simulink model "Batch_Model"  (Simulink 8.3)
settings: Solver=ode15s  StartTime=0.0  StopTime=10.0  RelTol=1e-2
values from neighbouring files (symbols this model uses):
  a0 = 555.556    [Ann_Main.m]    (also in Main_Program.m)
  B1 = 0.193    [Ann_Main.m]    (also in Main_Program.m)
  B2 = 0.167    [Ann_Main.m]    (also in Main_Program.m)
  c = S_Out    (= 0)    [Ann_Main.m]    (also in Main_Program.m = S_Out)
  c0 = 5.2*10^-5    (= 5.2e-05)    [Ann_Main.m]    (also in Main_Program.m)
  c1 = 16.4    [Ann_Main.m]    (also in Main_Program.m)
  c2 = 2.3    [Ann_Main.m]    (also in Main_Program.m)
  c3 = 1.563    [Ann_Main.m]    (also in Main_Program.m)
  CpC = 4.187    [Ann_Main.m]    (also in Main_Program.m)
  CpM = 1.675    [Ann_Main.m]    (also in Main_Program.m)
  CpP = 3.140    (= 3.14)    [Ann_Main.m]    (also in Main_Program.m)
  CpW = 4.187    [Ann_Main.m]    (also in Main_Program.m)
  d0 = 0.814    [Ann_Main.m]    (also in Main_Program.m)
  d1 = -5.13    [Ann_Main.m]    (also in Main_Program.m)
  deltaH = 70152.16    [Ann_Main.m]    (also in Main_Program.m)
  E = 29560.89    [Ann_Main.m]    (also in Main_Program.m)
  hf = 0.704    [Ann_Main.m]    (also in Main_Program.m = 0)
  i = 1.2    [Ann_Main.m]    (also in Main_Program.m)
  k0 = 55    [Ann_Main.m]    (also in Main_Program.m)
  k1 = 1000    [Ann_Main.m]    (also in Main_Program.m)
  k2 = 0.4    [Ann_Main.m]    (also in Main_Program.m)
  ki = 1    [Ann_Main.m]    (also in Main_Program.m = 0.8)
  mC = 21.455    [Ann_Main.m]    (also in Main_Program.m)
  mC_r = 0.9412    [Ann_Main.m]    (also in Main_Program.m)
  mMin = 0    [Ann_Main.m]    (also in Main_Program.m)
  mW = 42.750    (= 42.75)    [Ann_Main.m]    (also in Main_Program.m)
  MWM = 104.0    (= 104)    [Ann_Main.m]    (also in Main_Program.m)
  P = 1.594    [Ann_Main.m]    (also in Main_Program.m; S_ControllerPID.m = error-spid.error1)
  R = 8.314    [Ann_Main.m]    (also in Main_Program.m)
  rhoM = 900.0    (= 900)    [Ann_Main.m]    (also in Main_Program.m)
  rhoP = 1040.0    (= 1040)    [Ann_Main.m]    (also in Main_Program.m)
  rhoW = 1000.0    (= 1000)    [Ann_Main.m]    (also in Main_Program.m)
  TAmb = 305.38    [Ann_Main.m]    (also in Main_Program.m)
  tauP = 40.2    [Ann_Main.m]    (also in Main_Program.m)
  theta1 = 22.8    [Ann_Main.m]    (also in Main_Program.m)
  theta2 = 15    [Ann_Main.m]    (also in Main_Program.m)
  Tinlet = 294.26    [Ann_Main.m]    (also in Main_Program.m)
  TM = TAmb    (= 305.38)    [Ann_Main.m]    (also in Main_Program.m)
  Tsteam = 449.82    [Ann_Main.m]    (also in Main_Program.m)
  UAloss = 0.00567567    [Ann_Main.m]    (also in Main_Program.m)
settings Model: Creator=lijin  LastModifiedBy=Administrator
settings DataIOCC: ExternalInput=[k',mMin',c']
settings OptimizationCC: ExpressionDepthLimit=2147483647
settings DebuggingCC: FcnCallInpInsideContextMsg=UseLocalSettings

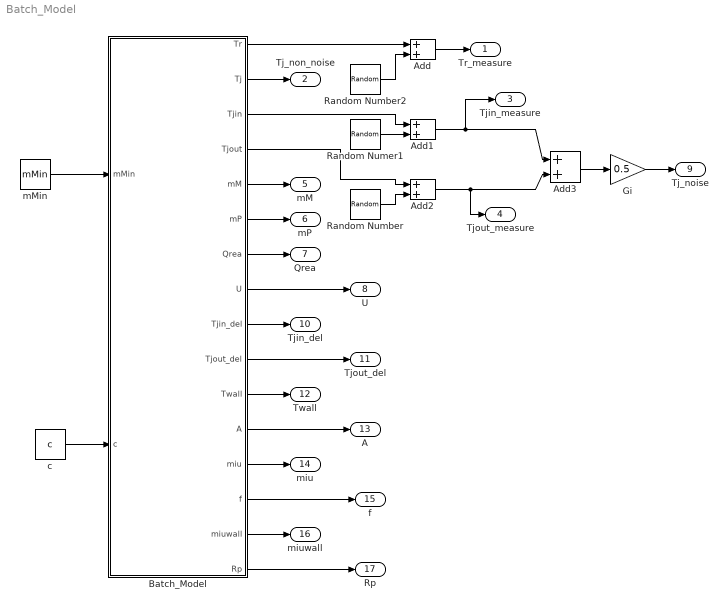
== system Batch_Model ==
  Add{,1..3} (4 alike) : Sum
  Batch_Model : Subsystem
  Gi : Gain  Gain=0.5
  Random Number : RandomNumber  Variance=0.01  Seed=34  SampleTime=0.1
  Random Number2 : RandomNumber  Variance=0.01  Seed=56  SampleTime=0.1
  Random Numer1 : RandomNumber  Variance=0.01  Seed=23  SampleTime=0.1
  c : Constant  Value=c  OutMin=[0]  OutMax=[100]  LockScale=on
  mMin : Constant  Value=mMin  OutMin=[0]  OutMax=[100]  LockScale=on
  Tr_measure : Outport
  Tj_non_noise : Outport  Port=2
  Tjin_measure : Outport  Port=3
  Tjout_measure : Outport  Port=4
  mM : Outport  Port=5
  mP : Outport  Port=6
  Qrea : Outport  Port=7
  U : Outport  Port=8
  Tj_noise : Outport  Port=9
  Tjin_del : Outport  Port=10
  Tjout_del : Outport  Port=11
  Twall : Outport  Port=12
  A : Outport  Port=13
  miu : Outport  Port=14
  f : Outport  Port=15
  miuwall : Outport  Port=16
  Rp : Outport  Port=17
  wires:
  mMin/1 -> Batch_Model/1(mMin)
  c/1 -> Batch_Model/2(c)
  Batch_Model/8(U) -> U/1
  Batch_Model/7(Qrea) -> Qrea/1
  Batch_Model/6(mP) -> mP/1
  Batch_Model/5(mM) -> mM/1
  Batch_Model/2(Tj) -> Tj_non_noise/1
  Batch_Model/3(Tjin) -> Add1/1
  Batch_Model/4(Tjout) -> Add2/1
  Random Numer1/1 -> Add1/2
  Random Number/1 -> Add2/2
  Batch_Model/1(Tr) -> Add/1
  Random Number2/1 -> Add/2
  Add/1 -> Tr_measure/1
  Add1/1 -> Tjin_measure/1, Add3/1
  Add2/1 -> Tjout_measure/1, Add3/2
  Add3/1 -> Gi/1
  Gi/1 -> Tj_noise/1
  Batch_Model/9(Tjin_del) -> Tjin_del/1
  Batch_Model/10(Tjout_del) -> Tjout_del/1
  Batch_Model/11(Twall) -> Twall/1
  Batch_Model/12(A) -> A/1
  Batch_Model/13(miu) -> miu/1
  Batch_Model/14(f) -> f/1
  Batch_Model/15(miuwall) -> miuwall/1
  Batch_Model/16(Rp) -> Rp/1

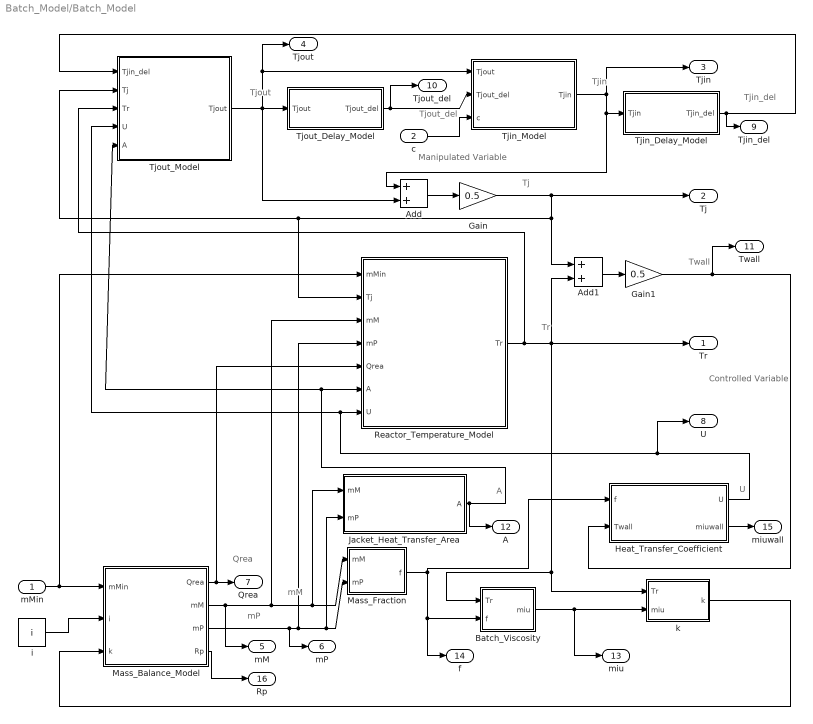
== system Batch_Model/Batch_Model ==
  note: Tj
  note: Tr
  note: Tjout
  note: Tjin
  note: Tjout_del
  note: Tjin_del
  note: U
  note: A
  note: mP
  note: mM
  note: Qrea
  note: Manipulated Variable
  note: Controlled Variable
  note: Twall
  mMin : Inport
  c : Inport  Port=2
  Add : Sum
  Add1 : Sum
  Batch_Viscosity : Subsystem
  Gain : Gain  Gain=0.5
  Gain1 : Gain  Gain=0.5
  Heat_Transfer_Coefficient : Subsystem
  Jacket_Heat_Transfer_Area : Subsystem
  Mass_Balance_Model : Subsystem
  Mass_Fraction : Subsystem
  Reactor_Temperature_Model : Subsystem
  Tjin_Delay_Model : Subsystem
  Tjin_Model : Subsystem
  Tjout_Delay_Model : Subsystem
  Tjout_Model : Subsystem
  i : Constant  Value=i
  k : Subsystem
  Tr : Outport
  Tj : Outport  Port=2
  Tjin : Outport  Port=3
  Tjout : Outport  Port=4
  mM : Outport  Port=5
  mP : Outport  Port=6
  Qrea : Outport  Port=7
  U : Outport  Port=8
  Tjin_del : Outport  Port=9
  Tjout_del : Outport  Port=10
  Twall : Outport  Port=11
  A : Outport  Port=12
  miu : Outport  Port=13
  f : Outport  Port=14
  miuwall : Outport  Port=15
  Rp : Outport  Port=16
  wires:
  Mass_Balance_Model/2(mM) -> Mass_Fraction/1(mM), Jacket_Heat_Transfer_Area/1(mM), Reactor_Temperature_Model/3(mM), mM/1
  Mass_Balance_Model/3(mP) -> Mass_Fraction/2(mP), Jacket_Heat_Transfer_Area/2(mP), Reactor_Temperature_Model/4(mP), mP/1
  Mass_Fraction/1(f) -> Batch_Viscosity/2(f), f/1, Heat_Transfer_Coefficient/1(f)
  Batch_Viscosity/1(miu) -> k/2(miu), miu/1
  Jacket_Heat_Transfer_Area/1(A) -> Reactor_Temperature_Model/6(A), Tjout_Model/5(A), A/1
  Heat_Transfer_Coefficient/1(U) -> Tjout_Model/4(U), Reactor_Temperature_Model/7(U), U/1
  Mass_Balance_Model/1(Qrea) -> Qrea/1, Reactor_Temperature_Model/5(Qrea)
  Tjout_Model/1(Tjout) -> Tjout_Delay_Model/1(Tjout), Tjout/1, Tjin_Model/1(Tjout), Add/2
  Tjout_Delay_Model/1(Tjout_del) -> Tjin_Model/2(Tjout_del), Tjout_del/1
  c/1 -> Tjin_Model/3(c)
  Tjin_Model/1(Tjin) -> Tjin_Delay_Model/1(Tjin), Add/1, Tjin/1
  Tjin_Delay_Model/1(Tjin_del) -> Tjout_Model/1(Tjin_del), Tjin_del/1
  Add/1 -> Gain/1
  Gain/1 -> Add1/1, Reactor_Temperature_Model/2(Tj), Tjout_Model/2(Tj), Tj/1
  mMin/1 -> Reactor_Temperature_Model/1(mMin), Mass_Balance_Model/1(mMin)
  Reactor_Temperature_Model/1(Tr) -> Tr/1, k/1(Tr), Batch_Viscosity/1(Tr), Add1/2, Tjout_Model/3(Tr)
  Add1/1 -> Gain1/1
  Gain1/1 -> Heat_Transfer_Coefficient/2(Twall), Twall/1
  Heat_Transfer_Coefficient/2(miuwall) -> miuwall/1
  Mass_Balance_Model/4(Rp) -> Rp/1
  i/1 -> Mass_Balance_Model/2(i)
  k/1(k) -> Mass_Balance_Model/3(k)

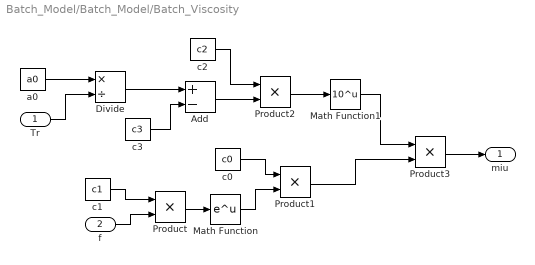
== system Batch_Model/Batch_Model/Batch_Viscosity ==
  Tr : Inport
  f : Inport  Port=2
  Add : Sum  Inputs=+-
  Divide : Product  Inputs=*/
  Math Function : Math  SaturateOnIntegerOverflow=on
  Math Function1 : Math  Operator=10^u  SaturateOnIntegerOverflow=on
  Product{,1..3} (4 alike) : Product  RndMeth=Zero
  a0 : Constant  Value=a0
  c0 : Constant  Value=c0
  c1 : Constant  Value=c1
  c2 : Constant  Value=c2
  c3 : Constant  Value=c3
  miu : Outport
  wires:
  c1/1 -> Product/1
  f/1 -> Product/2
  Product/1 -> Math Function/1
  Math Function/1 -> Product1/2
  c0/1 -> Product1/1
  a0/1 -> Divide/1
  Tr/1 -> Divide/2
  Divide/1 -> Add/1
  c3/1 -> Add/2
  Add/1 -> Product2/2
  c2/1 -> Product2/1
  Product2/1 -> Math Function1/1
  Math Function1/1 -> Product3/1
  Product1/1 -> Product3/2
  Product3/1 -> miu/1

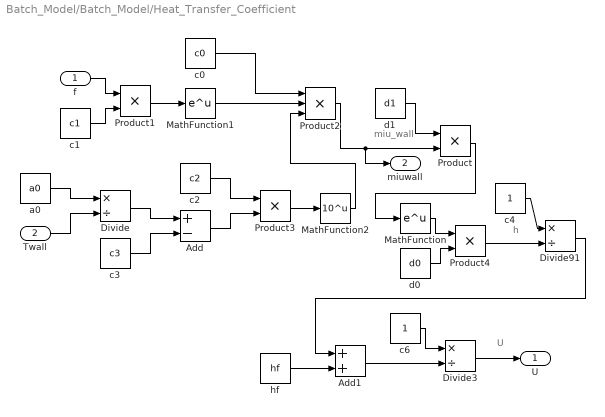
== system Batch_Model/Batch_Model/Heat_Transfer_Coefficient ==
  note: miu_wall
  note: h
  note: U
  f : Inport
  Twall : Inport  Port=2
  Add : Sum  Inputs=+-
  Add1 : Sum
  Divide : Product  Inputs=*/
  Divide3 : Product  Inputs=*/
  Divide91 : Product  Inputs=*/
  MathFunction : Math  SaturateOnIntegerOverflow=on
  MathFunction1 : Math  SaturateOnIntegerOverflow=on
  MathFunction2 : Math  Operator=10^u  SaturateOnIntegerOverflow=on
  Product{,1,3..4} (4 alike) : Product  RndMeth=Zero
  Product2 : Product  Inputs=3  RndMeth=Zero
  a0 : Constant  Value=a0
  c0 : Constant  Value=c0
  c1 : Constant  Value=c1
  c2 : Constant  Value=c2
  c3 : Constant  Value=c3
  c4 : Constant
  c6 : Constant
  d0 : Constant  Value=d0
  d1 : Constant  Value=d1
  hf : Constant  Value=hf
  U : Outport
  miuwall : Outport  Port=2
  wires:
  f/1 -> Product1/1
  c1/1 -> Product1/2
  Product1/1 -> MathFunction1/1
  a0/1 -> Divide/1
  Twall/1 -> Divide/2
  c3/1 -> Add/2
  Divide/1 -> Add/1
  Add/1 -> Product3/2
  c2/1 -> Product3/1
  Product3/1 -> MathFunction2/1
  c0/1 -> Product2/1
  MathFunction1/1 -> Product2/2
  MathFunction2/1 -> Product2/3
  Product2/1 -> Product/2, miuwall/1
  d1/1 -> Product/1
  MathFunction/1 -> Product4/1
  d0/1 -> Product4/2
  Product/1 -> MathFunction/1
  c4/1 -> Divide91/1
  Divide91/1 -> Add1/1
  c6/1 -> Divide3/1
  Add1/1 -> Divide3/2
  Divide3/1 -> U/1
  hf/1 -> Add1/2
  Product4/1 -> Divide91/2

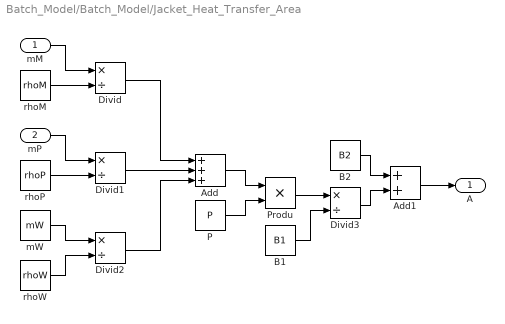
== system Batch_Model/Batch_Model/Jacket_Heat_Transfer_Area ==
  mM : Inport
  mP : Inport  Port=2
  Add : Sum  Inputs=+++
  Add1 : Sum
  B1 : Constant  Value=B1
  B2 : Constant  Value=B2
  Divid{,1..3} (4 alike) : Product  Inputs=*/
  P : Constant  Value=P
  Produ : Product  RndMeth=Zero
  mW : Constant  Value=mW
  rhoM : Constant  Value=rhoM
  rhoP : Constant  Value=rhoP
  rhoW : Constant  Value=rhoW
  A : Outport
  wires:
  mM/1 -> Divid/1
  rhoM/1 -> Divid/2
  mP/1 -> Divid1/1
  rhoP/1 -> Divid1/2
  mW/1 -> Divid2/1
  rhoW/1 -> Divid2/2
  Divid/1 -> Add/1
  Divid1/1 -> Add/2
  Divid2/1 -> Add/3
  Add/1 -> Produ/1
  P/1 -> Produ/2
  Produ/1 -> Divid3/1
  B1/1 -> Divid3/2
  B2/1 -> Add1/1
  Divid3/1 -> Add1/2
  Add1/1 -> A/1

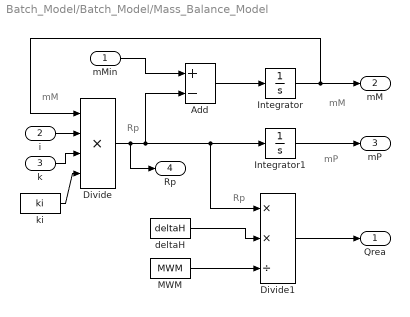
== system Batch_Model/Batch_Model/Mass_Balance_Model ==
  note: mM
  note: Rp
  note: Rp
  note: mM
  note: mP
  mMin : Inport
  i : Inport  Port=2
  k : Inport  Port=3
  Add : Sum  Inputs=+-
  Divide : Product  Inputs=****
  Divide1 : Product  Inputs=**/
  Integrator : Integrator
  Integrator1 : Integrator
  MWM : Constant  Value=MWM
  deltaH : Constant  Value=deltaH
  ki : Constant  Value=ki
  Qrea : Outport
  mM : Outport  Port=2
  mP : Outport  Port=3
  Rp : Outport  Port=4
  wires:
  i/1 -> Divide/2
  k/1 -> Divide/3
  mMin/1 -> Add/1
  Divide/1 -> Integrator1/1, Divide1/1, Add/2, Rp/1
  Add/1 -> Integrator/1
  Integrator/1 -> Divide/1, mM/1
  Integrator1/1 -> mP/1
  deltaH/1 -> Divide1/2
  Divide1/1 -> Qrea/1
  MWM/1 -> Divide1/3
  ki/1 -> Divide/4

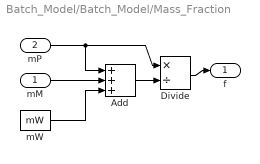
== system Batch_Model/Batch_Model/Mass_Fraction ==
  mM : Inport
  mP : Inport  Port=2
  Add : Sum  Inputs=+++
  Divide : Product  Inputs=*/
  mW : Constant  Value=mW
  f : Outport
  wires:
  mW/1 -> Add/3
  mM/1 -> Add/2
  mP/1 -> Add/1, Divide/1
  Add/1 -> Divide/2
  Divide/1 -> f/1

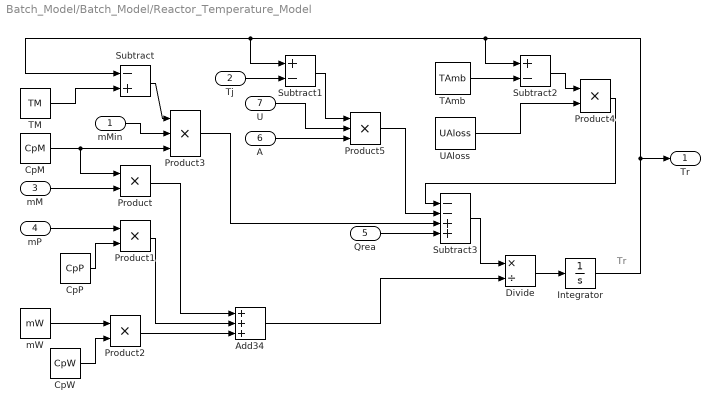
== system Batch_Model/Batch_Model/Reactor_Temperature_Model ==
  note: Tr
  mMin : Inport
  Tj : Inport  Port=2
  mM : Inport  Port=3
  mP : Inport  Port=4
  Qrea : Inport  Port=5
  A : Inport  Port=6
  U : Inport  Port=7
  Add34 : Sum  Inputs=+++
  CpM : Constant  Value=CpM
  CpP : Constant  Value=CpP
  CpW : Constant  Value=CpW
  Divide : Product  Inputs=*/
  Integrator : Integrator
  Product{,1..2,4} (4 alike) : Product  RndMeth=Zero
  Product3 : Product  Inputs=3  RndMeth=Zero
  Product5 : Product  Inputs=3  RndMeth=Zero
  Subtract : Sum  Inputs=-+
  Subtract1 : Sum  Inputs=+-
  Subtract2 : Sum  Inputs=+-
  Subtract3 : Sum  Inputs=--++
  TAmb : Constant  Value=TAmb
  TM : Constant  Value=TM
  UAloss : Constant  Value=UAloss
  mW : Constant  Value=mW
  Tr : Outport
  wires:
  mP/1 -> Product1/1
  CpP/1 -> Product1/2
  mW/1 -> Product2/1
  CpW/1 -> Product2/2
  Product/1 -> Add34/1
  Product1/1 -> Add34/2
  Product2/1 -> Add34/3
  mM/1 -> Product/2
  CpM/1 -> Product/1, Product3/3
  Tj/1 -> Subtract1/2
  mMin/1 -> Product3/2
  Subtract/1 -> Product3/1
  A/1 -> Product5/3
  U/1 -> Product5/2
  Subtract1/1 -> Product5/1
  TAmb/1 -> Subtract2/2
  Subtract2/1 -> Product4/1
  UAloss/1 -> Product4/2
  Integrator/1 -> Tr/1, Subtract/1, Subtract1/1, Subtract2/1
  Product4/1 -> Subtract3/1
  Product5/1 -> Subtract3/2
  Product3/1 -> Subtract3/3
  Qrea/1 -> Subtract3/4
  Subtract3/1 -> Divide/1
  Add34/1 -> Divide/2
  Divide/1 -> Integrator/1
  TM/1 -> Subtract/2

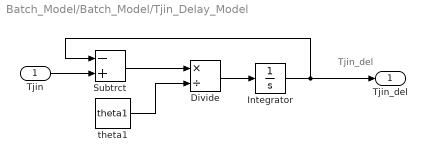
== system Batch_Model/Batch_Model/Tjin_Delay_Model ==
  note: Tjin_del
  Tjin : Inport
  Divide : Product  Inputs=*/
  Integrator : Integrator
  Subtrct : Sum  Inputs=-+
  theta1 : Constant  Value=theta1
  Tjin_del : Outport
  wires:
  Subtrct/1 -> Divide/1
  theta1/1 -> Divide/2
  Tjin/1 -> Subtrct/2
  Divide/1 -> Integrator/1
  Integrator/1 -> Tjin_del/1, Subtrct/1

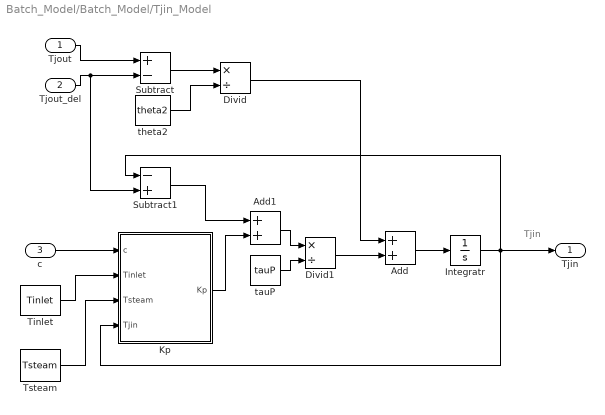
== system Batch_Model/Batch_Model/Tjin_Model ==
  note: Tjin
  Tjout : Inport
  Tjout_del : Inport  Port=2
  c : Inport  Port=3
  Add : Sum
  Add1 : Sum
  Divid : Product  Inputs=*/
  Divid1 : Product  Inputs=*/
  Integratr : Integrator
  Kp : MATLAB Function  TreatAsAtomicUnit=on
  Subtract : Sum  Inputs=+-
  Subtract1 : Sum  Inputs=-+
  Tinlet : Constant  Value=Tinlet
  Tsteam : Constant  Value=Tsteam
  tauP : Constant  Value=tauP
  theta2 : Constant  Value=theta2
  Tjin : Outport
  wires:
  Tjout/1 -> Subtract/1
  Tjout_del/1 -> Subtract/2, Subtract1/2
  Subtract/1 -> Divid/1
  theta2/1 -> Divid/2
  c/1 -> Kp/1(c)
  Tsteam/1 -> Kp/3(Tsteam)
  Integratr/1 -> Tjin/1, Subtract1/1, Kp/4(Tjin)
  Subtract1/1 -> Add1/1
  Add1/1 -> Divid1/1
  tauP/1 -> Divid1/2
  Divid/1 -> Add/1
  Divid1/1 -> Add/2
  Add/1 -> Integratr/1
  Kp/1(Kp) -> Add1/2
  Tinlet/1 -> Kp/2(Tinlet)

== system Batch_Model/Batch_Model/Tjout_Delay_Model ==
  note: Tjout_del
  Tjout : Inport
  Divide : Product  Inputs=*/
  Integrator : Integrator
  Subtrct : Sum  Inputs=-+
  theta2 : Constant  Value=theta2
  Tjout_del : Outport
  wires:
  Subtrct/1 -> Divide/1
  theta2/1 -> Divide/2
  Tjout/1 -> Subtrct/2
  Divide/1 -> Integrator/1
  Integrator/1 -> Tjout_del/1, Subtrct/1

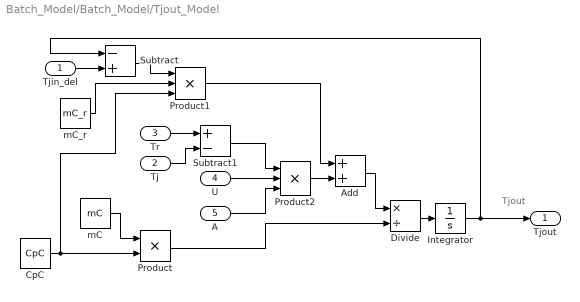
== system Batch_Model/Batch_Model/Tjout_Model ==
  note: Tjout
  Tjin_del : Inport
  Tj : Inport  Port=2
  Tr : Inport  Port=3
  U : Inport  Port=4
  A : Inport  Port=5
  Add : Sum
  CpC : Constant  Value=CpC
  Divide : Product  Inputs=*/
  Integrator : Integrator
  Product : Product  RndMeth=Zero
  Product1 : Product  Inputs=3  RndMeth=Zero
  Product2 : Product  Inputs=3  RndMeth=Zero
  Subtract : Sum  Inputs=-+
  Subtract1 : Sum  Inputs=+-
  mC : Constant  Value=mC
  mC_r : Constant  Value=mC_r
  Tjout : Outport
  wires:
  mC_r/1 -> Product1/2
  Tjin_del/1 -> Subtract/2
  Subtract/1 -> Product1/1
  Tr/1 -> Subtract1/1
  Tj/1 -> Subtract1/2
  Subtract1/1 -> Product2/1
  U/1 -> Product2/2
  A/1 -> Product2/3
  Product1/1 -> Add/1
  Product2/1 -> Add/2
  Product/1 -> Divide/2
  Add/1 -> Divide/1
  Divide/1 -> Integrator/1
  Integrator/1 -> Tjout/1, Subtract/1
  mC/1 -> Product/1
  CpC/1 -> Product/2, Product1/3

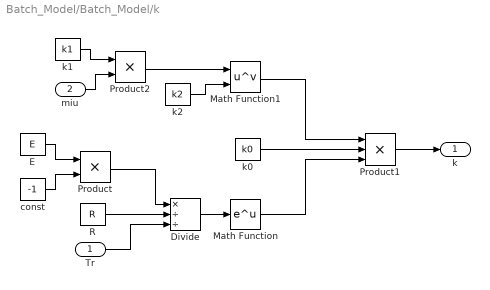
== system Batch_Model/Batch_Model/k ==
  Tr : Inport
  miu : Inport  Port=2
  Divide : Product  Inputs=*//
  E : Constant  Value=E
  Math Function : Math  SaturateOnIntegerOverflow=on
  Math Function1 : Math  Operator=pow  SaturateOnIntegerOverflow=on
  Product : Product  RndMeth=Zero
  Product1 : Product  Inputs=3  RndMeth=Zero
  Product2 : Product  RndMeth=Zero
  R : Constant  Value=R
  const : Constant  Value=-1
  k0 : Constant  Value=k0
  k1 : Constant  Value=k1
  k2 : Constant  Value=k2
  k : Outport
  wires:
  const/1 -> Product/2
  E/1 -> Product/1
  Product/1 -> Divide/1
  R/1 -> Divide/2
  Tr/1 -> Divide/3
  Divide/1 -> Math Function/1
  miu/1 -> Product2/2
  k1/1 -> Product2/1
  Product2/1 -> Math Function1/1
  k2/1 -> Math Function1/2
  k0/1 -> Product1/2
  Math Function/1 -> Product1/3
  Product1/1 -> k/1
  Math Function1/1 -> Product1/1

== matlab function Batch_Model/Tjin_Model/Kp ==
  data: c input double; Kp output double; Tinlet input double; Tsteam input double; Tjin input double
function Kp = fcn(c,Tinlet,Tsteam,Tjin)
if c>=0 && c<50
    Kp=0.8*30^(-c/50)*(Tinlet-Tjin);
elseif c==50
    Kp=0;
elseif c>50 && c<=100
    Kp=0.15*30^(c/50-2)*(Tsteam-Tjin);
else
    Kp=0;    
end
